simulink model "BMS_BalancingLogic_COM_Harness_SIL"  (R2022b)
settings: configuration reference "BMS_Sw_CodeGenConfig" (kept outside this file)
model workspace (MAT data in the model file):
  BATT.Manufacturer = 'Panasonic'
  BATT.Chemistry = 'Lithium Ion'
  BATT.Model = 'UR18650ZTA'
  BATT.Diameter = 18.24
  BATT.Length = 65.1
  BATT.CycleLife = 500
  BATT.Package.Ns_Module = 1
  BATT.Package.NumModules = 3
  BATT.Capacity.Rate = 2.85
  BATT.Capacity.Min = 2.9
  BATT.Capacity.Max = 3.1
  BATT.Capacity.MaxQ = 3.3046
  BATT.Capacity.Type = 3
  BATT.Res.R0 = 0.011333
  BATT.Res.R1 = 0.01
  BATT.Res.C1 = 0.003
  BATT.Res.R0_EOL = 0.0143
  BATT.Res.lambda = 1.066
  BATT.Voltage.Nominal = 3.7
  BATT.Voltage.NominalVolt = 3.4
  BATT.Voltage.Cut_off = 3
  BATT.Voltage.Init_Dchrg = 3.38
  BATT.Voltage.Full_Dchrg = 4.2
  BATT.Voltage.Max_Chrg = 4.35
  BATT.Voltage.V_LUT = [3 3.1 3.2 3.3 3.4 3.5 3.6 3.7 3.8 3.9 4 4.1 4.2]
  BATT.Temperature.Max = 50
  BATT.Temperature.Min = -20
  BATT.Temperature.Nominal = 20
  BATT.Temperature.dQ_dt = 0.005
  BATT.Temperature.T_LUT = [-20 -15 -10 -5 0 5 10 15 20 25 30 35 40 45 50]
  BATT.Temperature.derate_Fact = [0.599 0.6958 0.77 0.8246 0.87 0.913 0.95 0.981 1 1.005 1.01 1.018 1.03 1.057 1.1]
  BATT.Current.Dchrg = 6
  BATT.Current.Chrg = 1.45
  BATT.Current.Chrgfast = 2.5
  BATT.Current.threshold = 0.01
  BATT.SoC.SoC0 = 50
  BATT.SoC.max = 100
  BATT.SoC.min = 0
  BATT.SoC.alpha = 0.25
  BATT.SoC.Values = [0 10 20 30 40 50 60 70 80 90 100]
  BATT.SoC.iter = 10
  BATT.SoC.TableData = [20  10.6247  3.5915  0.7281  0.952  0.7379  0.4786  0.3427  0.2156  0.0885  0  0  0  0  0; 30  22.8077  14.7417  8.0781  1.2796  0.7453  0.486  0.3541  0.227  0.0999  0  0  0  0  0; 40  36.2545  27.8388  19.9116  11.9946  5.2721  0.4933  0.3655  0.2384  0.1113  0  0  0  0  0; 55  50.0995  41.4948  33.2185  24.9473  17.1653  9.4047  2.5769  0.1461  0.1227  0  0  0  0  0; 70  64.1003  55.36  46.9081  38.4492  30.311  22.1833  14.3739  7.0705  6.9056  6.7609  6.6376  6.5195  6.4218  6.3295; 85  77.975  69.3189  60.7318  52.1395  43.8339  35.5194  27.4362  19.6585  19.5776  19.5076  19.4494  19.3935  19.3492  19.3062; 90  89.649  83.1682  74.5397  65.9127  57.4716  49.0295  40.7915  32.8242  32.7783  32.7387  32.7064  32.6747  32.65  32.6259; 100  97.4996  94.2525  86.8985  79.671  71.1423  62.6136  54.2524  46.1531  46.1254  46.1016  46.0823  46.0631  46.0485  46.0339; 100  100  99.405  95.6128  91.9474  84.1242  76.2147  67.7605  59.5483  59.5317  59.5174  59.5056  59.4943  59.4853  59.4767; 100  100  100  100  98.3902  93.6674  89.1486  81.2168  72.969  72.9597  72.9518  72.9454  72.939  72.9341  72.9293; 100  100  100  100  100  99.6955  97.1736  92.8955  86.1238  86.1201  86.1168  86.1142  86.1117  86.1097  86.1077; 100  100  100  100  100  100  100  98.7573  95.7175  95.7169  95.7164  95.716  95.7157  95.7154  95.7151; 100  100  100  100  100  100  100  100  100  100  100  100  100  100  100]
  BATT.Balancing.Mode : BMS_BalMode_Enum (value not decoded)
  BATT.Balancing.ThresholdOn = 0.025
  BATT.Balancing.ThresholdOff = 0.01
  BATT.Balancing.BalWaitOff = 5
  BATT.Balancing.BalWaitOn = 10
  BATT.Balancing.Freq = 1000
  BATT.Balancing.Duty = 0.45
  BATT.InternalResistance = 0.04
  BATT.SOC_Init = 0.5
  BATT.LUT.SOC = [0 0.01 0.02 0.03 0.04 0.05 0.06 0.07 0.08 0.09 0.1 0.11 0.12 0.13 0.14 0.15 0.16 0.17 0.18 0.19 0.2 0.21 0.22 0.23 0.24 0.25 0.26 0.27 0.28 0.28999 0.3 0.31 0.32 0.33 0.34 0.35 0.36 0.37 0.38 0.39 0.4 0.41 0.42 0.43 0.44 0.45 0.46 0.47 0.48 0.49 0.5 0.51 0.52 0.53 0.54 0.55 0.56 0.56999 0.57999 0.59 0.6 0.61 0.62 0.63 0.64 0.65 0.66 0.67 0.68 0.69 0.7 0.71 0.72 0.73 0.74 0.75 0.76 0.77 0.78 0.79 0.8 0.81 0.82 0.83 0.84 0.85 0.86 0.87 0.88 0.89 0.9 0.91 0.92 0.93 0.94 0.95 0.96 0.97 0.98 0.99 1]
  BATT.LUT.T = [273.14999 298.14999 313.14999 333.14999]
  BATT.LUT.V0_T = [3.04339 3.19969 3.32733 3.41897 3.47789 3.5189 3.54757 3.56926 3.58543 3.59715 3.60656 3.61458 ... (404 elements, 101x4)]
  BATT.LUT.V0 = [3.04339 3.19969 3.32733 3.41897 3.47789 3.5189 3.54757 3.56926 3.58543 3.59715 3.60656 3.61458 3.62125 3.62859 3.63585 3.64117 3.64677 3.65281 3.65754 3.6622 3.66686 3.67118 3.67547 3.67953 3.68333 3.68679 3.68929 3.69163 3.69398 3.69633 3.69868 3.70108 3.7035 3.70592 3.70834 3.71076 3.71334 3.71599 3.71889 3.72198 3.72508 3.72817 3.73126 3.73436 3.73745 3.74054 3.74364 3.74686 3.75011 3.75346 3.75768 3.7621 3.76652 3.77094 3.77575 3.78058 3.78546 3.79147 3.79777 3.80409 3.8104 3.81672 3.82303 3.82935 3.83618 3.84344 3.8508 3.85816 3.86553 3.87289 3.88052 3.88833 3.89603 3.90423 3.91256 3.92124 3.93029 3.93933 3.94837 3.95788 3.96788 3.97854 3.98931 4.00007 4.01149 4.02304 4.03458 4.04614 4.05768 4.06947 4.08183 4.09422 4.1067 4.11982 4.1326 4.14614 4.15754 4.16699 4.17222 4.18119 4.30837]
  BATT.LUT.Vlim = [2.7 Inf]
  BATT.LUT.R0_T = [0.10009 0.14613 0.1823 0.20605 0.21852 0.22481 0.22685 0.22648 0.22421 0.2204 0.2158 0.21072 ... (404 elements, 101x4)]
  BATT.LUT.R0 = [0.04577 0.0693 0.0871 0.0981 0.10274 0.10473 0.1047 0.10401 0.1029 0.10084 0.09855 0.0961 0.09374 0.0923 0.09098 0.08942 0.08829 0.08779 0.08711 0.08642 0.08573 0.08504 0.08435 0.08362 0.08285 0.0821 0.08136 0.08067 0.07998 0.07929 0.07858 0.0779 0.07722 0.07655 0.07588 0.0752 0.07463 0.07414 0.07371 0.07333 0.07295 0.07256 0.07217 0.07179 0.07141 0.07102 0.07063 0.07034 0.07006 0.06981 0.06973 0.0697 0.06966 0.06963 0.06966 0.06969 0.06974 0.07 0.07016 0.07031 0.07047 0.07062 0.07078 0.07093 0.07117 0.07149 0.07185 0.07221 0.07256 0.07292 0.07332 0.07375 0.0741 0.07448 0.07489 0.07535 0.07584 0.07632 0.07682 0.07759 0.07865 0.07988 0.08112 0.08236 0.08368 0.08499 0.0863 0.08761 0.08891 0.09039 0.09225 0.09411 0.09597 0.09796 0.0995 0.10104 0.10043 0.09826 0.09216 0.08512 0.00997]
  BATT.LUT.SOC1 = [0 0.01 0.02 0.03 0.04 0.05 0.06 0.07 0.08 0.09 0.1 0.11 0.12 0.13 0.14 0.15 0.16 0.17 0.18 0.19 0.2 0.21 0.22 0.23 0.24 0.25 0.26 0.27 0.28 0.28999 0.3 0.31 0.32 0.33 0.34 0.35 0.36 0.37 0.38 0.39 0.4 0.41 0.42 0.43 0.44 0.45 0.46 0.47 0.48 0.49 0.5 0.51 0.52 0.53 0.54 0.55 0.56 0.56999 0.57999 0.59 0.6 0.61 0.62 0.63 0.64 0.65 0.66 0.67 0.68 0.69 0.7 0.71 0.72 0.73 0.74 0.75 0.76 0.77 0.78 0.79 0.8 0.81 0.82 0.83 0.84 0.85 0.86 0.87 0.88 0.89 0.9 0.91 0.92 0.93 0.94 0.95 0.96 0.97 0.98 0.99 1]
  BATT.LUT.R0D_T = [0.0117  0.0085  0.00899; 0.011  0.0085  0.00899; 0.0114  0.00869  0.0092; 0.0107  0.0082  0.0088; 0.0107  0.0083  0.0091; 0.0113  0.0085  0.0089; 0.0116  0.0085  0.0089]
  BATT.LUT.R0D = [0.0085 0.0085 0.00869 0.0082 0.0083 0.0085 0.0085]
  BATT.LUT.R0C_T = [0.0117  0.0085  0.00899; 0.011  0.0085  0.00899; 0.0114  0.00869  0.0092; 0.0107  0.0082  0.0088; 0.0107  0.0083  0.0091; 0.0113  0.0085  0.0089; 0.0116  0.0085  0.0089]
  BATT.LUT.R0C = [0.0085 0.0085 0.00869 0.0082 0.0083 0.0085 0.0085]
  Schedule.BMS_CurrentLimitsCalc_Task = 0.1
  Schedule.BMS_MainStateMachine_Task = 0.05
  Schedule.BMS_BalancingLogic_Task = 0.25
  Schedule.BMS_EstimateSOC_Task = 0.2
  Schedule.BMS_EstimateSOH_Task = 0.2
undefined symbols (not defined in the file): BMS_State_Enum
libraries: pil_lib x1
settings Model: DataDictionary=BMS_Arch_DD.sldd  Creator=MAAM  LastModifiedBy=MAAM
settings ConfigSetRef: SourceName=BMS_Sw_CodeGenConfig

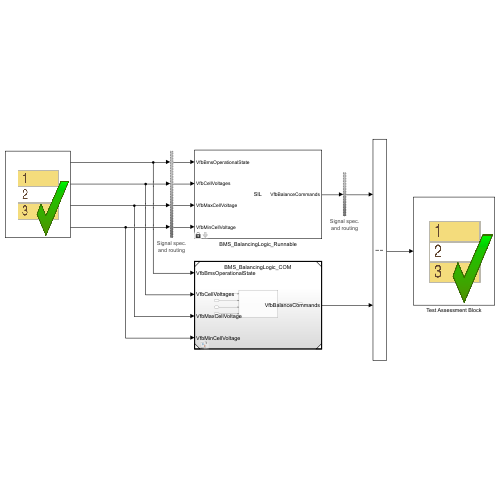
[thumbnail: Simulink's stored preview of the top-level diagram]
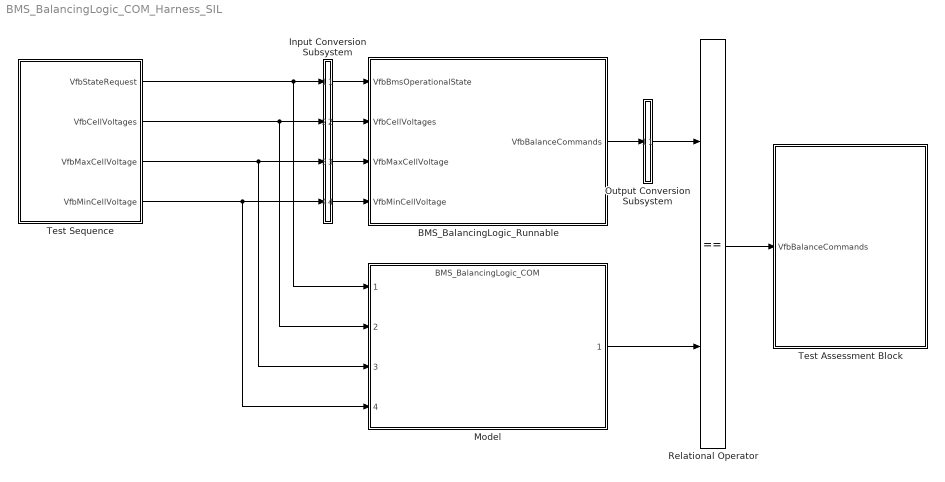
== system BMS_BalancingLogic_COM_Harness_SIL ==
  BMS_BalancingLogic_Runnable : Subsystem  Tag=__SL_testing_harness_stub_  DialogController=pil_create_dialog  LoadFcn=|
      | try
      |    if ~strcmp(rtw.pil.getPILVersion, '9.13 (R2022b)_15')
      |       set_param(gcb, 'DialogController', '');
      |       set_param(gcb, 'DialogControllerArgs', '');
      |    end
      | catch e
      |       set_param(gcb, 'DialogController', '');
      |       set_param(gcb, 'DialogControllerArgs', '');
      | end
      mask help: PIL:pil:XILBlockMaskDesc
      mask Display: disp('SIL');
  Input Conversion Subsystem : Subsystem  Tag=__SLT_ICS__  Description=|
      | Signal spec.
      | and routing
      settings: AttributesFormatString=%<Description>
  Model : ModelReference  ModelNameDialog=BMS_BalancingLogic_COM.slx  SimulationMode=Normal  ModelReferenceVersion=1.53
  Output Conversion Subsystem : Subsystem  Tag=__SLT_OCS__  Description=|
      | Signal spec.
      | and routing
      settings: AttributesFormatString=%<Description>
  Relational Operator : RelationalOperator  Operator===  OutDataTypeStr=boolean  RndMeth=Simplest  InputSameDT=off
  Test Assessment Block : Test Sequence  Tag=__SLT_ASMT__  TreatAsAtomicUnit=on
  Test Sequence : Test Sequence  TreatAsAtomicUnit=on
  wires:
  Test Sequence/1(VfbStateRequest) -> Model/1, Input Conversion Subsystem/1(Inport_1)
  Test Sequence/2(VfbCellVoltages) -> Model/2, Input Conversion Subsystem/2(Inport_2)
  Test Sequence/3(VfbMaxCellVoltage) -> Model/3, Input Conversion Subsystem/3(Inport_3)
  Test Sequence/4(VfbMinCellVoltage) -> Model/4, Input Conversion Subsystem/4(Inport_4)
  Relational Operator/1 -> Test Assessment Block/1(VfbBalanceCommands)
  Output Conversion Subsystem/1(Outport_1) -> Relational Operator/1
  Model/1 -> Relational Operator/2
  BMS_BalancingLogic_Runnable/1(VfbBalanceCommands) -> Output Conversion Subsystem/1(Inport_1)
  Input Conversion Subsystem/1(Outport_1) -> BMS_BalancingLogic_Runnable/1(VfbBmsOperationalState)
  Input Conversion Subsystem/2(Outport_2) -> BMS_BalancingLogic_Runnable/2(VfbCellVoltages)
  Input Conversion Subsystem/3(Outport_3) -> BMS_BalancingLogic_Runnable/3(VfbMaxCellVoltage)
  Input Conversion Subsystem/4(Outport_4) -> BMS_BalancingLogic_Runnable/4(VfbMinCellVoltage)

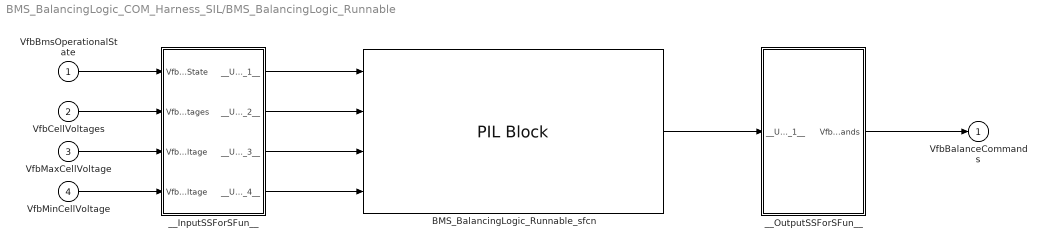
== system BMS_BalancingLogic_COM_Harness_SIL/BMS_BalancingLogic_Runnable ==
  VfbBmsOperationalState : Inport  OutDataTypeStr=Enum: BMS_State_Enum  PortDimensions=1
  VfbCellVoltages : Inport  Port=2
  VfbMaxCellVoltage : Inport  Port=3
  VfbMinCellVoltage : Inport  Port=4
  BMS_BalancingLogic_Runnable_sfcn : pil_lib/PIL Block  SimulationMode=SIL  IsTopModelPIL=off  CodeDir=BMS_BalancingLogic_Runnable_ert_rtw  AnchorDir=H:\0\New MAAM\10 - MBD\Battary Management System  ConfigName=Software-in-the-Loop (SIL)  XrelIsTopModelCode=on  XrelIsReusable=off  XrelDWorkNames={}  XrelDWorkTypes={}  XrelModelArgVals={}  XrelOrderedParamNames={}
  __InputSSForSFun__ : Subsystem
  __OutputSSForSFun__ : Subsystem
  VfbBalanceCommands : Outport
  wires:
  __OutputSSForSFun__/1(VfbBalanceCommands) -> VfbBalanceCommands/1
  BMS_BalancingLogic_Runnable_sfcn/1 -> __OutputSSForSFun__/1(__UniqueInportName__1__)
  __InputSSForSFun__/4(__UniqueOutportName__4__) -> BMS_BalancingLogic_Runnable_sfcn/4
  __InputSSForSFun__/3(__UniqueOutportName__3__) -> BMS_BalancingLogic_Runnable_sfcn/3
  __InputSSForSFun__/2(__UniqueOutportName__2__) -> BMS_BalancingLogic_Runnable_sfcn/2
  __InputSSForSFun__/1(__UniqueOutportName__1__) -> BMS_BalancingLogic_Runnable_sfcn/1
  VfbMinCellVoltage/1 -> __InputSSForSFun__/4(VfbMinCellVoltage)
  VfbMaxCellVoltage/1 -> __InputSSForSFun__/3(VfbMaxCellVoltage)
  VfbCellVoltages/1 -> __InputSSForSFun__/2(VfbCellVoltages)
  VfbBmsOperationalState/1 -> __InputSSForSFun__/1(VfbBmsOperationalState)

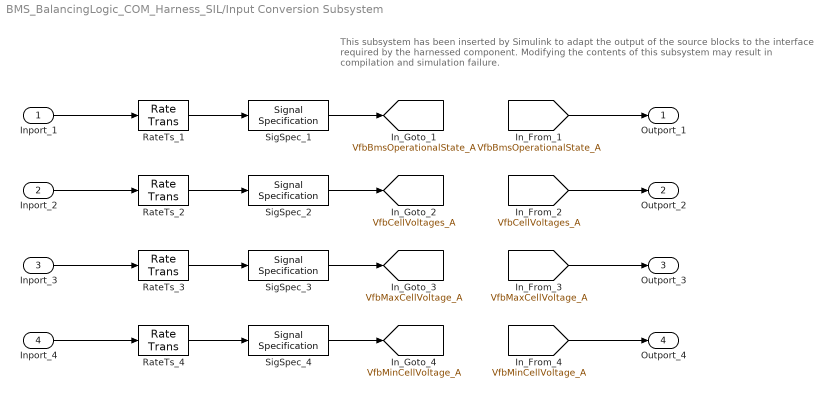
== system BMS_BalancingLogic_COM_Harness_SIL/Input Conversion Subsystem ==
  note: This subsystem has been inserted by Simulink to adapt the output of the source blocks to the interface required by the harnessed component.
      |  Modifying the contents of this subsystem may result in compilation and simulation failure.
  Inport_1 : Inport
  Inport_2 : Inport  Port=2
  Inport_3 : Inport  Port=3
  Inport_4 : Inport  Port=4
  RateTs_1 : RateTransition  InitialCondition=BMS_State_Enum.BMS_Standby  OutPortSampleTime=0.25
  RateTs_2 : RateTransition  OutPortSampleTime=0.25
  RateTs_3 : RateTransition  OutPortSampleTime=0.25
  RateTs_4 : RateTransition  OutPortSampleTime=0.25
  SigSpec_1 : SignalSpecification  OutDataTypeStr=Enum: BMS_State_Enum  Dimensions=[1]  SampleTime=0.25
  SigSpec_2 : SignalSpecification  OutDataTypeStr=single  Unit=V  Dimensions=[3]  SampleTime=0.25
  SigSpec_3 : SignalSpecification  OutDataTypeStr=single  Unit=V  Dimensions=[1]  SampleTime=0.25
  SigSpec_4 : SignalSpecification  OutDataTypeStr=single  Unit=V  Dimensions=[1]  SampleTime=0.25
  Outport_1 : Outport
  Outport_2 : Outport  Port=2
  Outport_3 : Outport  Port=3
  Outport_4 : Outport  Port=4
  tag scope: VfbBmsOperationalState_A=global, VfbCellVoltages_A=global, VfbMaxCellVoltage_A=global, VfbMinCellVoltage_A=global
  wires:
  [VfbBmsOperationalState_A] -> Outport_1/1
  SigSpec_1/1 -> [VfbBmsOperationalState_A]
  RateTs_1/1 -> SigSpec_1/1
  Inport_1/1 -> RateTs_1/1
  [VfbCellVoltages_A] -> Outport_2/1
  SigSpec_2/1 -> [VfbCellVoltages_A]
  RateTs_2/1 -> SigSpec_2/1
  Inport_2/1 -> RateTs_2/1
  [VfbMaxCellVoltage_A] -> Outport_3/1
  SigSpec_3/1 -> [VfbMaxCellVoltage_A]
  RateTs_3/1 -> SigSpec_3/1
  Inport_3/1 -> RateTs_3/1
  [VfbMinCellVoltage_A] -> Outport_4/1
  SigSpec_4/1 -> [VfbMinCellVoltage_A]
  RateTs_4/1 -> SigSpec_4/1
  Inport_4/1 -> RateTs_4/1

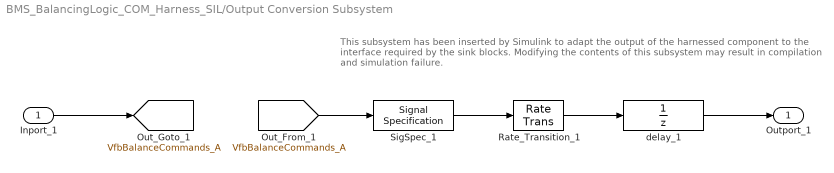
== system BMS_BalancingLogic_COM_Harness_SIL/Output Conversion Subsystem ==
  note: This subsystem has been inserted by Simulink to adapt the output of the harnessed component to the interface required by the sink blocks.
      |  Modifying the contents of this subsystem may result in compilation and simulation failure.
  Inport_1 : Inport
  Rate_Transition_1 : RateTransition  OutPortSampleTimeOpt=Inherit
  SigSpec_1 : SignalSpecification  OutDataTypeStr=boolean  Dimensions=[3]  SampleTime=0.25
  delay_1 : UnitDelay  SampleTime=-1
  Outport_1 : Outport
  tag scope: VfbBalanceCommands_A=global
  wires:
  Inport_1/1 -> [VfbBalanceCommands_A]
  [VfbBalanceCommands_A] -> SigSpec_1/1
  SigSpec_1/1 -> Rate_Transition_1/1
  Rate_Transition_1/1 -> delay_1/1
  delay_1/1 -> Outport_1/1

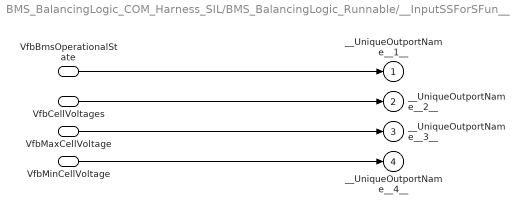
== system BMS_BalancingLogic_COM_Harness_SIL/BMS_BalancingLogic_Runnable/__InputSSForSFun__ ==
  VfbBmsOperationalState : Inport  OutDataTypeStr=Enum: BMS_State_Enum  PortDimensions=1
  VfbCellVoltages : Inport  Port=2
  VfbMaxCellVoltage : Inport  Port=3
  VfbMinCellVoltage : Inport  Port=4
  __UniqueOutportName__1__ : Outport
  __UniqueOutportName__2__ : Outport  Port=2
  __UniqueOutportName__3__ : Outport  Port=3
  __UniqueOutportName__4__ : Outport  Port=4
  wires:
  VfbMinCellVoltage/1 -> __UniqueOutportName__4__/1
  VfbMaxCellVoltage/1 -> __UniqueOutportName__3__/1
  VfbCellVoltages/1 -> __UniqueOutportName__2__/1
  VfbBmsOperationalState/1 -> __UniqueOutportName__1__/1

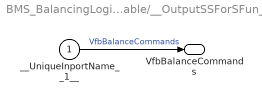
== system BMS_BalancingLogic_COM_Harness_SIL/BMS_BalancingLogic_Runnable/__OutputSSForSFun__ ==
  __UniqueInportName__1__ : Inport
  VfbBalanceCommands : Outport
  wires:
  __UniqueInportName__1__/1 -> VfbBalanceCommands/1  "VfbBalanceCommands"

== stateflow chart BMS_BalancingLogic_COM_Harness_SIL/Test Sequence ==
  settings: updateMethod=DISCRETE  sampleTime=0.25
  state Dynamic
    state Run
      VfbStateRequest = BMS_State_Enum.BMS_Balancing;
      VfbCellVoltages = single(3.7 * ones(3, 1));
      VfbMaxCellVoltage = single(3.7);
      VfbMinCellVoltage  = single(3.7);
    state S1
      VfbStateRequest = BMS_State_Enum.BMS_Balancing;
      VfbCellVoltages = single([3.725, 3.700, 3.700]');
      VfbMaxCellVoltage = single(3.725);
      VfbMinCellVoltage  = single(3.700);
    state S2
      VfbStateRequest = BMS_State_Enum.BMS_Balancing;
      VfbCellVoltages = single(3.7 * ones(3, 1));
      VfbMaxCellVoltage = single(3.7);
      VfbMinCellVoltage  = single(3.7);
    state S3
      VfbStateRequest = BMS_State_Enum.BMS_Balancing;
      VfbCellVoltages = single([3.725, 3.700, 3.700]');
      VfbMaxCellVoltage = single(3.725);
      VfbMinCellVoltage  = single(3.700);
    state S4
      VfbStateRequest = BMS_State_Enum.BMS_Driving;
      VfbCellVoltages = single([3.725, 3.700, 3.700]');
      VfbMaxCellVoltage = single(3.725);
      VfbMinCellVoltage  = single(3.700);
    state S5
      VfbStateRequest = BMS_State_Enum.BMS_Balancing;
      VfbCellVoltages = single([3.725, 3.700, 3.700]');
      VfbMaxCellVoltage = single(3.725);
      VfbMinCellVoltage  = single(3.700);
    state S6
      VfbStateRequest = BMS_State_Enum.BMS_Fault;
      VfbCellVoltages = single([3.725, 3.700, 3.700]');
      VfbMaxCellVoltage = single(3.725);
      VfbMinCellVoltage  = single(3.700);
    state S7
      VfbStateRequest = BMS_State_Enum.BMS_Standby;
      VfbCellVoltages = single([3.725, 3.700, 3.700]');
      VfbMaxCellVoltage = single(3.725);
      VfbMinCellVoltage  = single(3.700);
    state S8
      VfbStateRequest = BMS_State_Enum.BMS_Balancing;
      VfbCellVoltages = single([3.720, 3.700, 3.700]');
      VfbMaxCellVoltage = single(3.720);
      VfbMinCellVoltage  = single(3.700);
    state S9
      VfbStateRequest = BMS_State_Enum.BMS_Standby;
      VfbCellVoltages = single([3.725, 3.700, 3.700]');
      VfbMaxCellVoltage = single(3.725);
      VfbMinCellVoltage  = single(3.700);
    state S10
      VfbStateRequest = BMS_State_Enum.BMS_Standby;
      VfbCellVoltages = single([3.710, 3.700, 3.700]');
      VfbMaxCellVoltage = single(3.710);
      VfbMinCellVoltage  = single(3.700);
    state S11
      VfbStateRequest = BMS_State_Enum.BMS_Standby;
      VfbCellVoltages = single(3.7 * ones(3, 1));
      VfbMaxCellVoltage = single(3.7);
      VfbMinCellVoltage  = single(3.7);
    state S12
    state end
      coder.extrinsic('set_param');
      set_param(bdroot, 'SimulationCommand', 'stop');
    (default) -> Dynamic.Run
    Dynamic.Run -> Dynamic.S1 : [
        | after(1, sec)
        | ]
    Dynamic.S1 -> Dynamic.S2 : [
        | after(4.25, sec)
        | ]
    Dynamic.S2 -> Dynamic.S3 : [
        | after(9.75, sec)
        | ]
    Dynamic.S3 -> S4 : [
        | after(1, sec)
        | ]
    S4 -> S5 : [
        | after(1, sec)
        | ]
    S5 -> S6 : [
        | after(5, sec)
        | ]
    S6 -> S7 : [
        | after(1, sec)
        | ]
    S7 -> S8 : [
        | after(4.75, sec)
        | ]
    S8 -> S9 : [
        | after(1.25, sec)
        | ]
    S9 -> S10 : [
        | after(10, sec)
        | ]
    S10 -> S11 : [
        | after(5, sec)
        | ]
    S11 -> S12 : [
        | after(10, sec)
        | ]
    S12 -> Dynamic.end : [
        | after(5, sec)
        | ]
  state Ramp
    state Run
      VfbStateRequest = BMS_State_Enum.BMS_Balancing;
      VfbCellVoltages = single([3.725, 3.700, 3.700]');
      VfbMaxCellVoltage = single(3.725);
      VfbMinCellVoltage  = single(3.700);
    state S1
      VfbStateRequest = BMS_State_Enum.BMS_Balancing;
      VfbCellVoltages = single(3.4 + (4.2 - 3.4) * rand(3, 1));
      VfbMaxCellVoltage = max(VfbCellVoltages);
      VfbMinCellVoltage  =  min(VfbCellVoltages);
    state S2
      VfbCellVoltages = VfbCellVoltages - (VfbCellVoltages - VfbMinCellVoltage)  *ramp(et/5);
      VfbMaxCellVoltage = max(VfbCellVoltages);
      VfbMinCellVoltage  =  min(VfbCellVoltages);
    state S3
    state end
      coder.extrinsic('set_param');
      set_param(bdroot, 'SimulationCommand', 'stop');
    (default) -> Ramp.Run
    Ramp.Run -> Ramp.S1 : [
        | after(5, sec)
        | ]
    Ramp.S1 -> Ramp.S2 : [
        | after(1, sec)
        | ]
    Ramp.S2 -> Ramp.S1 [order 2] : [
        | after(5, sec)
        | ]
    Ramp.S2 -> Ramp.S3 [order 1] : [
        | t >(10*(1+5)+5)
        | ]
    Ramp.S3 -> Ramp.end : [
        | after(5, sec)
        | ]
  (default) -> Dynamic [order 1] : [Active_Scenario_Index == 1]
  (default) -> Ramp [order 2] : {assert(Active_Scenario_Index == 2,'The value of Scenario Parameter ''Active_Scenario_Index'' is not valid. Use the index of the scenario to specify it.')}
  data: VfbStateRequest output Enum: BMS_State_Enum size=[1]; VfbCellVoltages output single size=[3]; VfbMaxCellVoltage output single size=[1]; VfbMinCellVoltage output single size=[1]; Active_Scenario_Index parameter =1

== stateflow chart BMS_BalancingLogic_COM_Harness_SIL/Test Assessment Block ==
  state Run
    state step_1_1
      verify(all(VfbBalanceCommands == true));
    state step_1_2
    (default) -> (junction 22)
    Run -> (junction 22)
    (junction 22) -> (junction 23) [order 1] : [t > 5.5
        | ]
    (junction 23) -> step_1_1 [order 1] : [~in(Run.step_1_1)]
    (junction 22) -> (junction 31) [order 2]
    (junction 23) -> (junction 26) [order 2]
    (junction 31) -> (junction 32)
    (junction 32) -> step_1_2 [order 1] : [~in(Run.step_1_2)]
    (junction 32) -> (junction 35) [order 2]
  (default) -> Run
  data: VfbBalanceCommands input boolean size=[3]
